simulink model "lab1_q1_blockdiagram"  (Simulink 8.7)
settings: Solver=VariableStepAuto  StartTime=0.0  StopTime=5  RelTol=1e-3
settings Model: Creator=gmcma  LastModifiedBy=gmcma
settings DataIOCC: LimitDataPoints=off  SaveFormat=Dataset
settings DebuggingCC: UnderspecifiedInitializationDetection=Simplified  MergeDetectMultiDrivingBlocksExec=error
settings HardwareCC: ProdBitPerPointer=64  ProdLargestAtomicFloat=Float  ProdIntDivRoundTo=Zero  ProdEndianess=LittleEndian  ProdWordSize=64  ProdHWDeviceType=Intel->x86-64 (Windows64)
settings ModelReferenceCC: PropagateSignalLabelsOutOfModel=on
settings ConfigComp: CovModelRefEnable=off

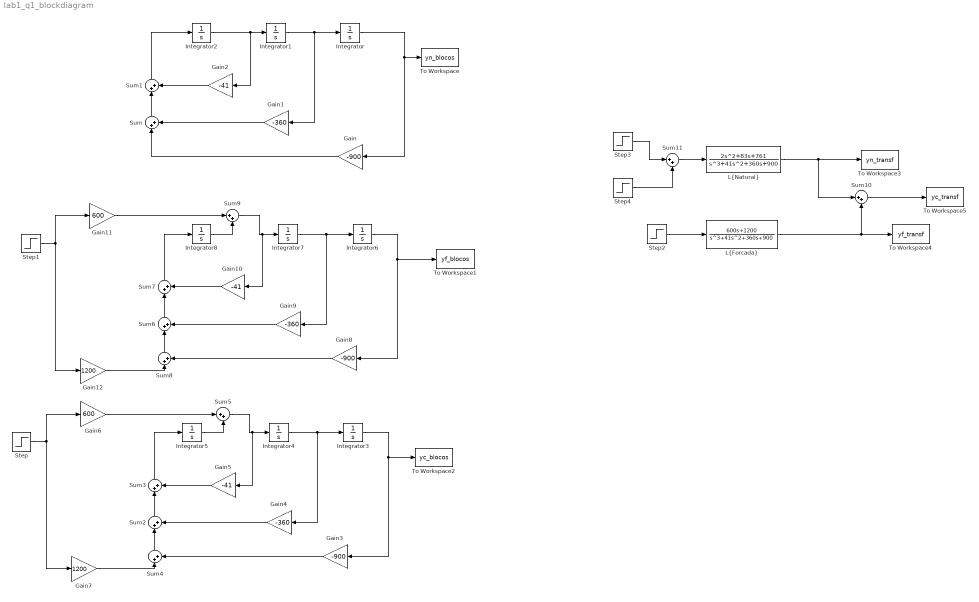
== system lab1_q1_blockdiagram ==
  Gain : Gain  Gain=-900
  Gain1 : Gain  Gain=-360
  Gain10 : Gain  Gain=-41
  Gain11 : Gain  Gain=600
  Gain12 : Gain  Gain=1200
  Gain2 : Gain  Gain=-41
  Gain3 : Gain  Gain=-900
  Gain4 : Gain  Gain=-360
  Gain5 : Gain  Gain=-41
  Gain6 : Gain  Gain=600
  Gain7 : Gain  Gain=1200
  Gain8 : Gain  Gain=-900
  Gain9 : Gain  Gain=-360
  Integrator : Integrator  InitialCondition=2
  Integrator1 : Integrator  InitialCondition=1
  Integrator2 : Integrator  InitialCondition=-0.05
  Integrator3 : Integrator  InitialCondition=2
  Integrator4 : Integrator  InitialCondition=1
  Integrator5 : Integrator  InitialCondition=-0.05
  Integrator6 : Integrator
  Integrator7 : Integrator
  Integrator8 : Integrator
  "L{Forcada}" : TransferFcn  Numerator=[600 1200]  Denominator=[1 41 360 900]
  "L{Natural}" : TransferFcn  Numerator=[2 83 761]  Denominator=[1 41 360 900]
  Step : Step  Time=0  SampleTime=0
  Step1 : Step  Time=0  SampleTime=0
  Step2 : Step  Time=0  SampleTime=0
  Step3 : Step  Time=0  After=100  SampleTime=0
  Step4 : Step  Time=0.01  After=-100  SampleTime=0
  Sum{,1..11} (12 alike) : Sum  Inputs=|++
  To Workspace : ToWorkspace  VariableName=yn_blocos  SaveFormat=Timeseries  SampleTime=-1
  To Workspace1 : ToWorkspace  VariableName=yf_blocos  SaveFormat=Timeseries  SampleTime=-1
  To Workspace2 : ToWorkspace  VariableName=yc_blocos  SaveFormat=Timeseries  SampleTime=-1
  To Workspace3 : ToWorkspace  VariableName=yn_transf  SaveFormat=Structure With Time  SampleTime=-1
  To Workspace4 : ToWorkspace  VariableName=yf_transf  SaveFormat=Structure With Time  SampleTime=-1
  To Workspace5 : ToWorkspace  VariableName=yc_transf  SaveFormat=Structure With Time  SampleTime=-1
  wires:
  Integrator1/1 -> Gain1/1, Integrator/1
  Integrator2/1 -> Gain2/1, Integrator1/1
  Integrator/1 -> To Workspace/1, Gain/1
  Gain1/1 -> Sum/2
  Gain/1 -> Sum/1
  Gain2/1 -> Sum1/2
  Sum/1 -> Sum1/1
  Sum1/1 -> Integrator2/1
  Integrator4/1 -> Gain4/1, Integrator3/1
  Integrator3/1 -> To Workspace2/1, Gain3/1
  Gain4/1 -> Sum2/2
  Gain5/1 -> Sum3/2
  Sum2/1 -> Sum3/1
  Sum3/1 -> Integrator5/1
  Step/1 -> Gain7/1, Gain6/1
  Gain7/1 -> Sum4/1
  Sum4/1 -> Sum2/1
  Gain3/1 -> Sum4/2
  Integrator5/1 -> Sum5/2
  Gain6/1 -> Sum5/1
  Sum5/1 -> Gain5/1, Integrator4/1
  Integrator7/1 -> Gain9/1, Integrator6/1
  Gain9/1 -> Sum6/2
  Gain10/1 -> Sum7/2
  Sum6/1 -> Sum7/1
  Sum7/1 -> Integrator8/1
  Step1/1 -> Gain12/1, Gain11/1
  Gain12/1 -> Sum8/1
  Sum8/1 -> Sum6/1
  Gain8/1 -> Sum8/2
  Integrator8/1 -> Sum9/2
  Gain11/1 -> Sum9/1
  Sum9/1 -> Gain10/1, Integrator7/1
  Integrator6/1 -> To Workspace1/1, Gain8/1
  Sum10/1 -> To Workspace5/1
  "L{Forcada}"/1 -> To Workspace4/1, Sum10/2
  "L{Natural}"/1 -> To Workspace3/1, Sum10/1
  Step2/1 -> "L{Forcada}"/1
  Step3/1 -> Sum11/1
  Step4/1 -> Sum11/2
  Sum11/1 -> "L{Natural}"/1
